simulink model "PizzaBox"  (R2018b)
settings: Solver=FixedStepAuto  StartTime=0.0  StopTime=inf  RelTol=1e-3  EnableMultiTasking=on
undefined symbols (not defined in the file or in its folder): dev, Main, pwm_output0
libraries: aerolibutil x7, px4Sensorslib x4, px4uORBlib x3, simulink x2, px4lib x1, sharedtransform x1
(part 1 of 2)
settings Model: xpc_rtwmakecfg_data=_xpcnblib_  SimulationMode=external  ExtModeTrigDuration=10  Creator=Robert  LastModifiedBy=Robert
settings SolverCC: PositivePriorityOrder=on
settings DataIOCC: SaveOutput=off  SignalLogging=off  DSMLogging=off  SaveTime=off
settings OptimizationCC: DefaultUnderspecifiedDataType=single  EnhancedBackFolding=on  PassReuseOutputArgsAs=Individual arguments  MaxStackSize=64  OptimizeBlockOrder=speed  DifferentSizesBufferReuse=on  OptimizationCustomize=off
settings DebuggingCC: ParameterTunabilityLossMsg=error
settings HardwareCC: ProdBitPerPointer=32  ProdBitPerSizeT=32  ProdBitPerPtrDiffT=32  ProdLargestAtomicInteger=Long  ProdLargestAtomicFloat=Double  ProdWordSize=32  ProdLongLongMode=on  ProdHWDeviceType=ARM Compatible->ARM Cortex
settings SFSimCC: MATLABDynamicMemAlloc=off
settings RTWCC: SystemTargetFile=ert.tlc  HardwareBoard=PX4 Pixhawk 1  TLCOptions="-aInlineSetEventsForThisBaseRateFcn=TLC_FALSE -aSuppressMultiTaskScheduler=TLC_FALSE  -aRateBasedStepFcn=0"  TemplateMakefile=ert_default_tmf  GenerateReport=on  Toolchain=GNU Tools for PX4 Autopilots  IncludeHyperlinkInReport=on  LaunchReport=on  TargetLang=C++  GenerateTraceInfo=on  GenerateTraceReport=on  GenerateTraceReportSl=on  GenerateTraceReportSf=on  GenerateTraceReportEml=on
settings CodeAppCC: ForceParamTrailComments=on  IgnoreCustomStorageClasses=off  OperatorAnnotations=on  SimulinkDataObjDesc=on  SFDataObjDesc=on  InsertBlockDesc=on
settings ERTTargetCC: ExtMode=on  ExtModeMexArgs='127.0.0.1' 1 17725

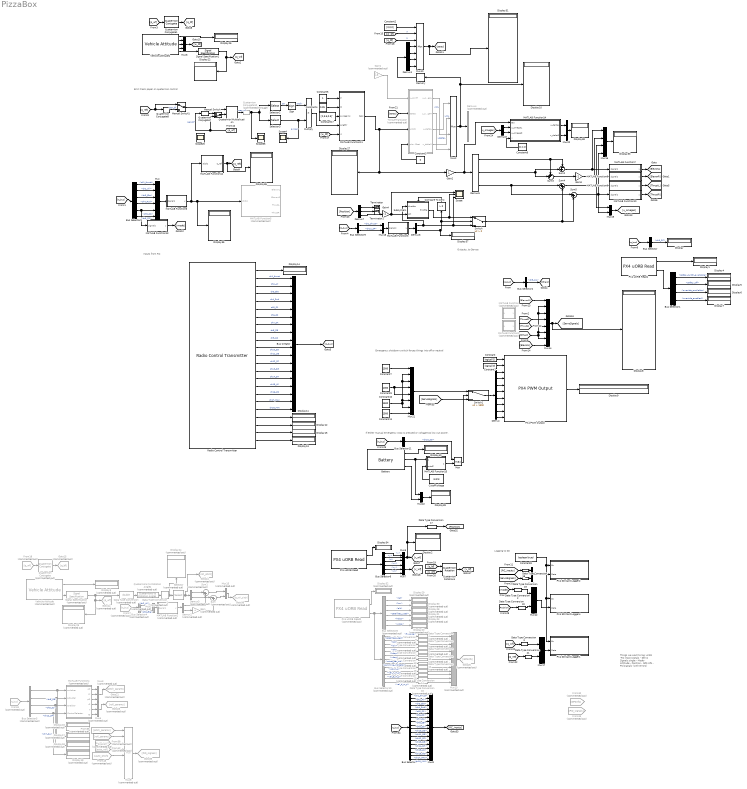
== system PizzaBox ==
  note: If either manual emergency stop is pressed or voltage too low cut power.
  note: Emergency shutdown switch forces things into
      | off or neutral
  note: Logging to SD
  note: Inputs from RC
  note: Outputs, to Servos
  note: Things we want to log:
      |
      | uint8
      | -RC input signals
      | - Servo Signals
      |
      | single
      | - Mode
      | - Attitude
      | - Position
      | - GPS info
      | - Pid signals (with errors)
  note: Emil Fresk paper on quaternion control
  Battery : px4Sensorslib/Battery  voltage=on  current=off  remaining=on  warning=off  timestamp=off  sampleTime=1/250  BlockingMode=off  BlockTimeout=1e-3
      settings: SourceProductName=Embedded Coder Support Package for PX4 Autopilots
  Bus Creator : BusCreator  Inputs=18
  Bus Selector : BusSelector  OutputSignals=ch9_SC
  Bus Selector1 : BusSelector  OutputSignals=safety_switch_available,safety_off,override_available,override_enabled
  Bus Selector10 : BusSelector  Commented=on  OutputSignals=fix_type,satellites_used,lat,lon,alt,hdop,vdop,noise_per_ms,jamming_indicator,vel_m_s,vel_n_m_s,vel_e_m_s,vel_d_m_s
  Bus Selector11 : BusSelector  OutputSignals=ch10_SD
  Bus Selector2 : BusSelector  OutputSignals=ch5_S1
  Bus Selector3 : BusSelector  OutputSignals=ch1_thrust,ch2_Ail,ch3_Ele,ch4_Rud,ch9_SC,ch6_S2
  Bus Selector4 : BusSelector  Commented=on  OutputSignals=ch2_Ail,ch3_Ele
  Bus Selector5 : BusSelector  Commented=on  OutputSignals=ch8_SB,ch5_S1,ch12_SF,ch7_SA
  Bus Selector6 : BusSelector  OutputSignals=x,y,z,vx,vy,vz
  Bus Selector7 : BusSelector  OutputSignals=ch1_thrust,ch2_Ail,ch3_Ele,ch4_Rud,ch5_S1,ch6_S2,ch7_SA,ch8_SB,ch9_SC,ch10_SD,ch11_SE,ch12_SF,ch13_SG,ch14_SH,ch15_LS,ch16_RS,ch17_MAX,ch18_MIN
  Bus Selector8 : BusSelector  Commented=on  OutputSignals=lat,lon,alt,satellites_used,hdop,vdop
  Bus Selector9 : BusSelector  OutputSignals=ch1_thrust,ch12_SF
  Compare To Zero : simulink/Logic and Bit Operations/Compare To Zero  relop=>  OutDataTypeStr=boolean
  Constant : Constant  Value=logical(1)
  Constant1 : Constant  Value=logical(0)
  Constant10 : Constant  Value=1500  OutDataTypeStr=uint16
  Constant11 : Constant  Value=1500  OutDataTypeStr=uint16
  Constant17 : Constant  Value=[2,3.5,0.3]'  VectorParams1D=off
  Constant2 : Constant  Value=[0,0,0]  OutDataTypeStr=single
  Constant3 : Constant  Value=0
  Constant4 : Constant  Value=0.25
  Constant5 : Constant
  Constant6 : Constant  Value=[0,0,0]
  Constant7 : Constant  Value=1500  OutDataTypeStr=uint16
  Constant8 : Constant  Value=boolean(true)  OutDataTypeStr=boolean  SampleTime=0.004
  Constant9 : Constant  Value=1000  OutDataTypeStr=uint16
  CutoffVoltage : Constant  Value=3.3*3  OutDataTypeStr=single
  Data Type Conversion : DataTypeConversion  Commented=on  OutDataTypeStr=double
  Data Type Conversion{1,4..16} (14 alike) : DataTypeConversion  Commented=on  OutDataTypeStr=single
  Data Type Conversion{2..3,17,20..21} (5 alike) : DataTypeConversion  OutDataTypeStr=single
  Data Type Conversion18 : DataTypeConversion  OutDataTypeStr=uint16
  Data Type Conversion19 : DataTypeConversion  OutDataTypeStr=uint16
  Demux : Demux  Outputs=8
  Demux1 : Demux
  Demux2 : Demux  Commented=on  Outputs=2
  Demux3 : Demux  Commented=on  Outputs=2
  Demux4 : Demux  Commented=on
  Demux5 : Demux  Outputs=3
  Demux6 : Demux  Outputs=2
  Demux7 : Demux  Outputs=3
  Demux8 : Demux  Outputs=2
  Display{,1..2,4..15,22,26..27,31,33..40} (27 alike) : Display
      Display9 settings: Format=binary (Stored Integer)
  Display{3,16..21,23..25,28..30,32} (14 alike) : Display  Commented=on
  From18 : From  Commented=on  GotoTag=q_wf
  From30 : From  Commented=on  GotoTag=GPSinfo
  From33 : From  Commented=on  GotoTag=PID_signals
  From36 : From  Commented=on  GotoTag=pitch_params
  From37 : From  Commented=on  GotoTag=roll_params
  From38 : From  Commented=on  GotoTag=e_roll_pitch
  From42 : From  Commented=on  GotoTag=auto_roll
  From43 : From  Commented=on  GotoTag=auto_pitch
  From7 : From  Commented=on  GotoTag=rc_bus
  From8 : From  Commented=on  GotoTag=rc_bus
  Gain : Gain  Commented=on  Gain=-1
  Gain1 : Gain  Commented=on  Gain=18
  Gain2 : Gain
  Gain3 : Gain  Gain=-1
  Gain4 : Gain  Gain=-1
  Goto14 : Goto  Commented=on  GotoTag=q_wf
  Goto15 : Goto  Commented=on  GotoTag=q_bf
  Goto21 : Goto  Commented=on  GotoTag=pitch_params
  Goto23 : Goto  Commented=on  GotoTag=roll_params
  Goto24 : Goto  Commented=on  GotoTag=roll_pitch
  Goto25 : Goto  Commented=on  GotoTag=GPSinfo
  Goto35 : Goto  Commented=on  GotoTag=PID_signals
  Goto36 : Goto  Commented=on  GotoTag=e_roll_pitch
  MATLAB Function : MATLAB Function  Commented=on  TreatAsAtomicUnit=on
  MATLAB Function1 : MATLAB Function  Commented=on  TreatAsAtomicUnit=on
  MATLAB Function10 : MATLAB Function  TreatAsAtomicUnit=on
  MATLAB Function11 : MATLAB Function  TreatAsAtomicUnit=on
  MATLAB Function12 : MATLAB Function  TreatAsAtomicUnit=on
  MATLAB Function13 : MATLAB Function  TreatAsAtomicUnit=on
  MATLAB Function14 : MATLAB Function  TreatAsAtomicUnit=on
  MATLAB Function15 : MATLAB Function  TreatAsAtomicUnit=on
  MATLAB Function2 : MATLAB Function  Commented=on  TreatAsAtomicUnit=on
  MATLAB Function3 : MATLAB Function  TreatAsAtomicUnit=on
  MATLAB Function4 : MATLAB Function  Commented=on  TreatAsAtomicUnit=on
  MATLAB Function5 : MATLAB Function  Commented=on  TreatAsAtomicUnit=on
  MATLAB Function6 : MATLAB Function  TreatAsAtomicUnit=on
  MATLAB Function7 : MATLAB Function  TreatAsAtomicUnit=on
  MATLAB Function8 : MATLAB Function  TreatAsAtomicUnit=on
  MATLAB Function9 : MATLAB Function  TreatAsAtomicUnit=on
  Manual Switch : ManualSwitch  CurrentSetting=0
  Manual Switch1 : ManualSwitch
  Max : MinMax  Function=max  Inputs=2  OutDataTypeStr=uint16
  Memory : Memory
  Multiply : Product
  Mux : Mux  Inputs=6
  Mux1 : Mux  Commented=on  Inputs=2
  Mux10 : Mux  Inputs=7
  Mux{11..12,17..20,22} (7 alike) : Mux  Inputs=2
  Mux13 : Mux  Commented=on  Inputs=13
  Mux14 : Mux  Inputs=8
  Mux15 : Mux  Commented=on  Inputs=2
  Mux16 : Mux
  Mux2 : Mux
  Mux21 : Mux  Inputs=8
  Mux3 : Mux  Commented=on  Inputs=3
  Mux4 : Mux  Commented=on  Inputs=3
  Mux5 : Mux  Inputs=3
  Mux6 : Mux  Inputs=3
  Mux7 : Mux  Inputs=3
  Mux8 : Mux  Inputs=18
  Mux9 : Mux  Commented=on  Inputs=8
  PX4 PWM Output : px4lib/PX4 PWM Output  pwmDevice=Main (/dev/pwm_output0)  pwmChannel1_=on  pwmChannel2_=on  pwmChannel3_=on  pwmChannel4_=on  pwmChannel5_=on  pwmChannel6_=on  pwmChannel7_=on  pwmChannel8_=on  forceTerminateFailsafe=off  outputErrorStatus=on
      settings: SourceProductName=Embedded Coder Support Package for PX4 Autopilots
  PX4 SD Card Logger1 : Subsystem  mask(PX4 SD Card Logger){logfile=/fs/microsd/log, logfilename=qlogs, cacheflag=off, numRecs=250*60*60}
      mask prompts: logfile "Log Folder"; logfilename "Log File Name"; cacheflag "Cache in Memory"; numRecs "Maximum Record Count"
      mask help:
      | Log data to a specified file on the SD card
      |
      | The block accepts two inputs, enable and data. The incoming data is logged into the SD card when the enable signal is high and the number of data points logged is less than the Maximum Record Count specified.
      |
      | The specified folder should be present in the SD card for logging.
      |
      | If Cache in Memory is unchecked, the data is written to the SD card at every timestep.  If Cache in Memory is checked, data is cached in the memory and is written to SD card only when enable goes low or when the number of data points logged reaches the Maximum Record Count specified.
      mask init:
      | logname=uint8([logfile,'/',logfilename]);
      mask Help: eval('codertarget.internal.helpView(''px4'',''px4sdcardexample'')');
      mask Display:
      | fprintf([get_param(gcb,'logfile'),'/',get_param(gcb,'logfilename')])
      | port_label('input',1,'en')
      | port_label('input',2,'data')
  PX4 SD Card Logger2 : Subsystem  mask(PX4 SD Card Logger){logfile=/fs/microsd/log, logfilename=rc_and_servosignals, cacheflag=off, numRecs=250*60*60}
      mask prompts: logfile "Log Folder"; logfilename "Log File Name"; cacheflag "Cache in Memory"; numRecs "Maximum Record Count"
      mask help:
      | Log data to a specified file on the SD card
      |
      | The block accepts two inputs, enable and data. The incoming data is logged into the SD card when the enable signal is high and the number of data points logged is less than the Maximum Record Count specified.
      |
      | The specified folder should be present in the SD card for logging.
      |
      | If Cache in Memory is unchecked, the data is written to the SD card at every timestep.  If Cache in Memory is checked, data is cached in the memory and is written to SD card only when enable goes low or when the number of data points logged reaches the Maximum Record Count specified.
      mask init:
      | logname=uint8([logfile,'/',logfilename]);
      mask Help: eval('codertarget.internal.helpView(''px4'',''px4sdcardexample'')');
      mask Display:
      | fprintf([get_param(gcb,'logfile'),'/',get_param(gcb,'logfilename')])
      | port_label('input',1,'en')
      | port_label('input',2,'data')
  PX4 SD Card Logger4 : Subsystem  mask(PX4 SD Card Logger){logfile=/fs/microsd/log, logfilename=MainLog, cacheflag=off, numRecs=250*60*60}
      mask prompts: logfile "Log Folder"; logfilename "Log File Name"; cacheflag "Cache in Memory"; numRecs "Maximum Record Count"
      mask help:
      | Log data to a specified file on the SD card
      |
      | The block accepts two inputs, enable and data. The incoming data is logged into the SD card when the enable signal is high and the number of data points logged is less than the Maximum Record Count specified.
      |
      | The specified folder should be present in the SD card for logging.
      |
      | If Cache in Memory is unchecked, the data is written to the SD card at every timestep.  If Cache in Memory is checked, data is cached in the memory and is written to SD card only when enable goes low or when the number of data points logged reaches the Maximum Record Count specified.
      mask init:
      | logname=uint8([logfile,'/',logfilename]);
      mask Help: eval('codertarget.internal.helpView(''px4'',''px4sdcardexample'')');
      mask Display:
      | fprintf([get_param(gcb,'logfile'),'/',get_param(gcb,'logfilename')])
      | port_label('input',1,'en')
      | port_label('input',2,'data')
  PX4 uORB Read : px4uORBlib/PX4 uORB Read  uORBTopic=vehicle_local_position  sampleTime=0.004  BlockingMode=off  BlockTimeout=1e-3
      settings: SourceProductName=Embedded Coder Support Package for PX4 Autopilots
  PX4 uORB Read1 : px4uORBlib/PX4 uORB Read  uORBTopic=safety  sampleTime=0.004  BlockingMode=off  BlockTimeout=1e-3
      settings: SourceProductName=Embedded Coder Support Package for PX4 Autopilots
  PX4 uORB Read2 : px4uORBlib/PX4 uORB Read  Commented=on  uORBTopic=vehicle_gps_position  sampleTime=0.004  BlockingMode=off  BlockTimeout=1e-3
      settings: SourceProductName=Embedded Coder Support Package for PX4 Autopilots
  Quaternion Conjugate : aerolibutil/Quaternion Conjugate  Commented=on
      settings: SourceProductName=Aerospace Blockset  SourceProductBaseCode=AE
  Quaternion Conjugate1 : aerolibutil/Quaternion Conjugate
      settings: SourceProductName=Aerospace Blockset  SourceProductBaseCode=AE
  Quaternion Conjugate10 : aerolibutil/Quaternion Conjugate  Commented=through
      settings: SourceProductName=Aerospace Blockset  SourceProductBaseCode=AE
  Quaternion Conjugate7 : aerolibutil/Quaternion Conjugate
      settings: SourceProductName=Aerospace Blockset  SourceProductBaseCode=AE
  Quaternion Conjugate8 : aerolibutil/Quaternion Conjugate
      settings: SourceProductName=Aerospace Blockset  SourceProductBaseCode=AE
  Quaternion Multiplication : aerolibutil/Quaternion Multiplication
  Quaternion Rotation4 : aerolibutil/Quaternion Rotation
  Quaternions to Rotation Angles : sharedtransform/Quaternions to Rotation Angles  Commented=on  rotationOrder=ZYX  aMode=aMode
      settings: SourceProductBaseCode=AE
  Radio Control Transmitter : px4Sensorslib/Radio Control Transmitter  channel1=on  channel2=on  channel3=on  channel4=on  channel5=on  channel6=on  channel7=on  channel8=on  channel9=on  channel10=on  channel11=on  channel12=on  channel13=on  channel14=on  channel15=on  channel16=on  channel17=on  channel18=on  channel_count=on  rssi=on  rc_input_source=on  timestamp_last_signal=on  time_stamp=off  sampleTime=1/250  BlockingMode=off  BlockTimeout=5
      settings: SourceProductName=Embedded Coder Support Package for PX4 Autopilots
  Scope : Scope  NumInputPorts=3
  Scope25 : Scope
  Scope35 : Scope
  Scope4 : Scope
  Selector : Selector  Commented=on  InputPortWidth=3  IndexOptions=Index vector (dialog)  Indices=[3 2]  OutputSizes=1
  Selector2 : Selector  IndexMode=Zero-based  InputPortWidth=4  IndexOptions=Index vector (dialog)  Indices=[0 ]  OutputSizes=1
  Selector3 : Selector  IndexMode=Zero-based  InputPortWidth=4  IndexOptions=Index vector (dialog)  Indices=[1:3]  OutputSizes=1
  Sign : Signum
  Signal Specification : SignalSpecification  Commented=on  OutDataTypeStr=single
  Signal Specification1 : SignalSpecification  OutDataTypeStr=single
  Subsystem : Subsystem
  Sum : Sum  Commented=on  Inputs=|-+
  Sum1 : Sum  Commented=on  Inputs=|-+
  Sum2 : Sum  Inputs=-+|
  Sum3 : Sum  Inputs=++|
  Sum4 : Sum  Inputs=|++
  Sum5 : Sum  Inputs=|-+
  Switch : Switch  Criteria=u2 > Threshold
  Switch1 : Switch  Criteria=u2 > Threshold  Threshold=1300
  Terminator : Terminator
  Terminator1 : Terminator
  TorqueTranslator : MATLAB Function  Commented=on  TreatAsAtomicUnit=on
  Vehicle Attitude : px4Sensorslib/Vehicle Attitude  Commented=on  rollRate=off  pitchRate=off  yawRate=off  quaternion=on  uorbTimeStamp=off  BlockingMode=off  BlockTimeout=0.001  sampleTime=1/250
      settings: SourceProductName=Embedded Coder Support Package for PX4 Autopilots
  Vehicle Attitude1 : px4Sensorslib/Vehicle Attitude  rollRate=on  pitchRate=on  yawRate=on  quaternion=on  uorbTimeStamp=off  BlockingMode=off  BlockTimeout=0.001  sampleTime=1/250
      settings: SourceProductName=Embedded Coder Support Package for PX4 Autopilots
  wires:
  Vehicle Attitude/2 -> Signal Specification/1
  Vehicle Attitude/1 -> Display3/1
  Radio Control Transmitter/8 -> Bus Creator/7  "ch7_SA"
  Radio Control Transmitter/7 -> Bus Creator/6  "ch6_S2"
  Radio Control Transmitter/6 -> Bus Creator/5  "ch5_S1"
  Radio Control Transmitter/2 -> Bus Creator/1  "ch1_thrust"
  Radio Control Transmitter/3 -> Bus Creator/2  "ch2_Ail"
  Radio Control Transmitter/4 -> Bus Creator/3  "ch3_Ele"
  Radio Control Transmitter/5 -> Bus Creator/4  "ch4_Rud"
  Radio Control Transmitter/9 -> Bus Creator/8  "ch8_SB"
  Radio Control Transmitter/20 -> Display11/1
  Radio Control Transmitter/21 -> Display12/1
  Radio Control Transmitter/23 -> Display13/1
  Radio Control Transmitter/1 -> Display14/1
  Radio Control Transmitter/22 -> Display15/1
  Constant/1 -> PX4 PWM Output/1
  Constant1/1 -> PX4 PWM Output/2
  Bus Creator/1 -> [rc_bus]
  Quaternions to Rotation Angles/1 -> Data Type Conversion1/1
  Bus Selector/1 -> Display/1  "<ch9_SC>"
  Demux3/1 -> Sum1/1
  Demux3/2 -> Sum/1
  Signal Specification/1 -> Goto14/1, Display25/1, Data Type Conversion/1
  [rc_bus] -> Bus Selector2/1
  [rc_bus] -> Bus Selector/1
  Bus Selector2/1 -> [Others]  "<ch5_S1>"
  Data Type Conversion/1 -> Quaternions to Rotation Angles/1
  Demux2/2 -> Gain/1
  From7/1 -> Bus Selector4/1
  Bus Selector4/1 -> Mux1/1  "<ch2_Ail>"
  Bus Selector4/2 -> Mux1/2  "<ch3_Ele>"
  Mux1/1 -> MATLAB Function2/1(signals)
  MATLAB Function2/1(y) -> Demux2/1
  Demux2/1 -> Sum1/2
  Mux4/1 -> Goto23/1
  From8/1 -> Bus Selector5/1
  Bus Selector5/2 -> Display17/1, MATLAB Function4/2(adjuster)  "<ch5_S1>"
  Bus Selector5/1 -> Display16/1, MATLAB Function4/1(switcher)  "<ch8_SB>"
  MATLAB Function4/1(pP) -> Mux3/1
  MATLAB Function4/2(pI) -> Mux3/2
  MATLAB Function4/3(pD) -> Mux3/3
  Bus Selector5/3 -> Display18/1, MATLAB Function4/3(enabler)  "<ch12_SF>"
  Radio Control Transmitter/10 -> Bus Creator/9  "ch9_SC"
  Radio Control Transmitter/11 -> Bus Creator/10  "ch10_SD"
  Radio Control Transmitter/12 -> Bus Creator/11  "ch11_SE"
  Radio Control Transmitter/13 -> Bus Creator/12  "ch12_SF"
  Radio Control Transmitter/14 -> Bus Creator/13  "ch13_SG"
  Radio Control Transmitter/15 -> Bus Creator/14  "ch14_SH"
  Radio Control Transmitter/16 -> Bus Creator/15  "ch15_LS"
  Radio Control Transmitter/17 -> Bus Creator/16  "ch16_RS"
  Radio Control Transmitter/18 -> Bus Creator/17  "ch17_MAX"
  Radio Control Transmitter/19 -> Bus Creator/18  "ch18_MIN"
  MATLAB Function4/4(rP) -> Mux4/1
  MATLAB Function4/5(rI) -> Mux4/2
  MATLAB Function4/6(rD) -> Mux4/3
  Bus Selector5/4 -> Display19/1, MATLAB Function4/4(ControlSelector)  "<ch7_SA>"
  PX4 uORB Read/2 -> Bus Selector6/1
  PX4 uORB Read2/2 -> Bus Selector10/1, Bus Selector8/1
  PX4 uORB Read/1 -> Display34/1
  PX4 uORB Read2/1 -> Display32/1
  Bus Selector6/1 -> Mux5/1  "<x>"
  Bus Selector6/2 -> Mux5/2  "<y>"
  Bus Selector6/3 -> Mux5/3  "<z>"
  Bus Selector8/1 -> Display29/1  "<lat>"
  Bus Selector8/2 -> Display30/1  "<lon>"
  Bus Selector8/3 -> Display28/1  "<alt>"
  Sum1/1 -> Mux15/1
  Sum/1 -> Mux15/2
  Gain/1 -> Sum/2
  Mux3/1 -> Goto21/1
  Selector/1 -> Goto24/1, Demux3/1
  Mux5/1 -> Data Type Conversion17/1, Display2/1, [r_wf]
  From18/1 -> Quaternion Conjugate/1
  Quaternion Conjugate/1 -> Goto15/1
  Bus Selector6/4 -> Mux7/1  "<vx>"
  Bus Selector6/5 -> Mux7/2  "<vy>"
  Bus Selector6/6 -> Mux7/3  "<vz>"
  Mux7/1 -> [v_wf]
  Quaternion Rotation4/1 -> [v_bf]
  [v_wf] -> Quaternion Rotation4/2
  [q_bf] -> Quaternion Rotation4/1
  Bus Selector8/4 -> Display21/1  "<satellites_used>"
  Bus Selector8/5 -> Display23/1  "<hdop>"
  Bus Selector8/6 -> Display20/1  "<vdop>"
  Data Type Conversion1/1 -> Display24/1, Selector/1
  Constant8/1 -> PX4 SD Card Logger1/1(En), PX4 SD Card Logger4/1(En), PX4 SD Card Logger2/1(En)
  Mux11/1 -> PX4 SD Card Logger2/2(Data)
  [RC_inputs] -> Data Type Conversion18/1
  [ServoSignals] -> Data Type Conversion19/1
  Mux12/1 -> PX4 SD Card Logger4/2(Data)
  [mode] -> Data Type Conversion2/1
  [Position] -> Data Type Conversion20/1
  Bus Selector10/1 -> Data Type Conversion4/1  "<fix_type>"
  Bus Selector10/2 -> Data Type Conversion5/1  "<satellites_used>"
  Bus Selector10/3 -> Data Type Conversion6/1  "<lat>"
  Bus Selector10/4 -> Data Type Conversion7/1  "<lon>"
  Bus Selector10/5 -> Data Type Conversion8/1  "<alt>"
  Bus Selector10/6 -> Data Type Conversion9/1  "<hdop>"
  Bus Selector10/7 -> Data Type Conversion10/1  "<vdop>"
  Bus Selector10/8 -> Data Type Conversion11/1  "<noise_per_ms>"
  Bus Selector10/9 -> Data Type Conversion12/1  "<jamming_indicator>"
  Bus Selector10/10 -> Data Type Conversion13/1  "<vel_m_s>"
  Bus Selector10/11 -> Data Type Conversion14/1  "<vel_n_m_s>"
  Bus Selector10/12 -> Data Type Conversion15/1  "<vel_e_m_s>"
  Bus Selector10/13 -> Data Type Conversion16/1  "<vel_d_m_s>"
  Mux13/1 -> Goto25/1
  [rc_bus] -> Bus Selector7/1
  Bus Selector7/1 -> Mux8/1  "<ch1_thrust>"
  Bus Selector7/2 -> Mux8/2  "<ch2_Ail>"
  Bus Selector7/3 -> Mux8/3  "<ch3_Ele>"
  Bus Selector7/4 -> Mux8/4  "<ch4_Rud>"
  Bus Selector7/5 -> Mux8/5  "<ch5_S1>"
  Bus Selector7/6 -> Mux8/6  "<ch6_S2>"
  Bus Selector7/7 -> Mux8/7  "<ch7_SA>"
  Bus Selector7/8 -> Mux8/8  "<ch8_SB>"
  Bus Selector7/9 -> Mux8/9  "<ch9_SC>"
  Bus Selector7/10 -> Mux8/10  "<ch10_SD>"
  Bus Selector7/11 -> Mux8/11  "<ch11_SE>"
  Bus Selector7/12 -> Mux8/12  "<ch12_SF>"
  Bus Selector7/13 -> Mux8/13  "<ch13_SG>"
  Bus Selector7/14 -> Mux8/14  "<ch14_SH>"
  Bus Selector7/15 -> Mux8/15  "<ch15_LS>"
  Bus Selector7/16 -> Mux8/16  "<ch16_RS>"
  Bus Selector7/17 -> Mux8/17  "<ch17_MAX>"
  Bus Selector7/18 -> Mux8/18  "<ch18_MIN>"
  Mux8/1 -> [RC_inputs]
  Mux14/1 -> Display8/1, [ServoSignals]
  Demux/1 -> PX4 PWM Output/3
  Demux/2 -> PX4 PWM Output/4
  Demux/3 -> PX4 PWM Output/5
  Demux/4 -> PX4 PWM Output/6
  Demux/5 -> PX4 PWM Output/7
  Demux/6 -> PX4 PWM Output/8
  Demux/7 -> PX4 PWM Output/9
  Demux/8 -> PX4 PWM Output/10
  Mux9/1 -> Goto35/1
  From36/1 -> Mux9/1
  From37/1 -> Mux9/2
  Mux15/1 -> Goto36/1
  From38/1 -> Mux9/3
  Data Type Conversion4/1 -> Mux13/1
  Data Type Conversion5/1 -> Mux13/2
  Data Type Conversion6/1 -> Mux13/3
  Data Type Conversion7/1 -> Mux13/4
  Data Type Conversion8/1 -> Mux13/5
  Data Type Conversion9/1 -> Mux13/6
  Data Type Conversion10/1 -> Mux13/7
  Data Type Conversion11/1 -> Mux13/8
  Data Type Conversion12/1 -> Mux13/9
  Data Type Conversion13/1 -> Mux13/10
  Data Type Conversion14/1 -> Mux13/11
  Data Type Conversion15/1 -> Mux13/12
  Data Type Conversion16/1 -> Mux13/13
  Data Type Conversion17/1 -> [Position]
  Data Type Conversion18/1 -> Mux11/1
  Data Type Conversion19/1 -> Mux11/2
  From42/1 -> Mux9/4
  From43/1 -> Mux9/5
  [ThrustR] -> Mux14/4
  [ThrustL] -> Mux14/5
  [ElevonR] -> Mux14/1
  [ElevonL] -> Mux14/8
  [Others] -> Mux14/2, Mux14/3, Mux14/6, Mux14/7
  [rc_bus] -> Bus Selector3/1
  Bus Selector3/4 -> Mux/4  "<ch4_Rud>"
  Bus Selector3/1 -> Mux/1  "<ch1_thrust>"
  Bus Selector3/3 -> Mux/3  "<ch3_Ele>"
  Bus Selector3/2 -> Mux/2  "<ch2_Ail>"
  Mux/1 -> MATLAB Function6/1(signals)
  MATLAB Function6/1(y) -> MATLAB Function12/1(sticks), Display35/1, MATLAB Function5/1(sticks)
  MATLAB Function7/1(y) -> [ElevonL]
  MATLAB Function8/1(y) -> [ElevonR]
  MATLAB Function9/1(y) -> [ThrustL]
  MATLAB Function10/1(y) -> [ThrustR]
  PX4 uORB Read1/1 -> Display1/1
  PX4 uORB Read1/2 -> Bus Selector1/1
  Bus Selector1/1 -> Display4/1  "<safety_switch_available>"
  Bus Selector1/2 -> Display5/1  "<safety_off>"
  Bus Selector1/3 -> Display6/1  "<override_available>"
  Bus Selector1/4 -> Display7/1  "<override_enabled>"
  PX4 PWM Output/1 -> Display9/1
  Signal Specification1/1 -> [q_wf], Display22/1
  [q_wf] -> Quaternion Conjugate1/1
  Quaternion Conjugate1/1 -> [q_bf]
  Vehicle Attitude1/1 -> Display26/1
  Vehicle Attitude1/5 -> Signal Specification1/1
  Vehicle Attitude1/2 -> Mux6/1
  Vehicle Attitude1/3 -> Mux6/2
  Vehicle Attitude1/4 -> Mux6/3
  Mux6/1 -> [w_bf]
  Sign/1 -> Multiply/1  "rotdir"
  [w_bf] -> MATLAB Function11/5(w)
  Quaternion Multiplication/1 -> Quaternion Conjugate10/1  "qerr_wf"
  Quaternion Conjugate10/1 -> Selector3/1, Selector2/1, Scope35/1
  Constant17/1 -> MATLAB Function11/3(axisgains)
  Selector3/1 -> Multiply/2, Scope4/1  "axiserr"
  [q_wf] -> Manual Switch/2, Quaternion Conjugate7/1  "qerr_bf"
  Multiply/1 -> MATLAB Function11/4(angErr)
  Selector2/1 -> Sign/1  "q0"
  [q_ref] -> Manual Switch1/1, Quaternion Conjugate8/1
  Constant2/1 -> Mux10/1
  [w_bf] -> Mux10/2  "w"
  [q_bf] -> Mux10/3  "q"
  MATLAB Function12/1(q_ref) -> Display36/1, [q_ref]
  Demux1/1 -> Mux10/4
  Demux1/2 -> Mux10/5
  Demux1/3 -> Mux10/6
  Demux1/4 -> Mux10/7
  Memory/1 -> Demux1/1
  TorqueTranslator/3(u_deltaL) -> Mux2/1  "uWL"
  TorqueTranslator/4(u_deltaR) -> Mux2/2  "udeltaL"
  TorqueTranslator/2(u_omegaR) -> Mux2/4
  TorqueTranslator/1(u_omegaL) -> Mux2/3  "uWL"
  Mux10/1 -> Display31/1, [states]
  [states] -> TorqueTranslator/2(states)
  Constant3/1 -> TorqueTranslator/4(pitchoffset)
  MATLAB Function11/1(taos) -> Gain2/1, Display27/1, TorqueTranslator/3(wdots)
  Gain1/1 -> TorqueTranslator/1(u_jointT)
  Mux2/1 -> Display10/1, Memory/1, Demux4/1
  Sum3/1 -> Gain3/1
  Sum4/1 -> Mux19/1, Mux16/3, MATLAB Function9/1(signals)
  Sum5/1 -> Mux19/2, Mux16/4, MATLAB Function10/1(signals)
  Bus Selector9/1 -> Mux18/1  "<ch1_thrust>"
  Switch/1 -> Sum4/2, Sum5/2
  [rc_bus] -> Bus Selector9/1
  Demux5/3 -> Sum5/1, Sum4/1
  Gain2/1 -> Demux5/1, MATLAB Function14/1(tao)
  Constant5/1 -> MATLAB Function11/1(P)
  Constant4/1 -> MATLAB Function11/2(D)
  Sum2/1 -> Mux16/1, MATLAB Function7/1(signals)
  Mux16/1 -> Display33/1
  Quaternion Conjugate7/1 -> Manual Switch/1
  Manual Switch/1 -> Quaternion Multiplication/2
  Quaternion Conjugate8/1 -> Manual Switch1/2  "qerr_bf"
  Manual Switch1/1 -> Quaternion Multiplication/1
  Demux5/2 -> Sum3/2, Sum2/2
  Demux5/1 -> Sum2/1, Sum3/1
  Gain3/1 -> Mux16/2, MATLAB Function8/1(signals)
  Bus Selector3/5 -> MATLAB Function13/1(signals), Mux/5  "<ch9_SC>"
  Bus Selector3/6 -> Mux/6  "<ch6_S2>"
  MATLAB Function13/1(y) -> [mode]
  Data Type Conversion2/1 -> Mux12/1
  Data Type Conversion20/1 -> Mux12/2
  [q_ref] -> Data Type Conversion21/1
  [q_wf] -> Data Type Conversion3/1
  Data Type Conversion3/1 -> Mux17/1
  Data Type Conversion21/1 -> Mux17/2
  Mux17/1 -> PX4 SD Card Logger1/2(Data)
  Bus Selector9/2 -> Mux18/2  "<ch12_SF>"
  Mux18/1 -> MATLAB Function3/1(signals)
  MATLAB Function3/1(y) -> Demux6/1
  Demux6/2 -> Display37/1, Switch/2, Compare To Zero/1
  Demux6/1 -> Subsystem/1(throttle), Scope/3, Switch/3
  [Position] -> Demux7/1
  Demux7/1 -> Terminator/1
  Demux7/2 -> Terminator1/1
  Demux7/3 -> Gain4/1
  Gain4/1 -> Scope/1, Subsystem/2(alt)
  Compare To Zero/1 -> Subsystem/Enable
  Subsystem/1("throttle ") -> Scope/2, Switch/1
  Constant6/1 -> MATLAB Function14/4(v)
  Mux19/1 -> [u_omegas]
  Demux8/1 -> MATLAB Function14/2(u_omegaL)
  Demux8/2 -> MATLAB Function14/3(u_omegaR)
  [u_omegas] -> Demux8/1
  MATLAB Function14/2(u_deltaR) -> Mux20/2
  MATLAB Function14/1(u_deltaL) -> Mux20/1
  Mux20/1 -> Display38/1
  [rc_bus] -> Bus Selector11/1
  Max/1 -> Switch1/2
  [ServoSignals] -> Switch1/3
  Constant10/1 -> Mux21/2, Mux21/3, Mux21/6, Mux21/7
  Constant9/1 -> Mux21/4, Mux21/5
  Constant11/1 -> Mux21/8
  Constant7/1 -> Mux21/1
  Mux21/1 -> Switch1/1
  Switch1/1 -> Demux/1
  MATLAB Function15/1(stopsig) -> Max/2
  Bus Selector11/1 -> Max/1  "<ch10_SD>"
  Battery/2 -> MATLAB Function15/1(voltage), Mux22/1
  Battery/3 -> Mux22/2
  Mux22/1 -> Display39/1
  Battery/1 -> Display40/1
  CutoffVoltage/1 -> MATLAB Function15/2(cutoff)

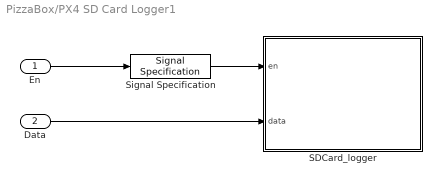
== system PizzaBox/PX4 SD Card Logger1 ==
  En : Inport
  Data : Inport  Port=2
  SDCard_logger : MATLAB Function  TreatAsAtomicUnit=on
  Signal Specification : SignalSpecification  OutDataTypeStr=boolean
  wires:
  Signal Specification/1 -> SDCard_logger/1(en)
  En/1 -> Signal Specification/1
  Data/1 -> SDCard_logger/2(data)

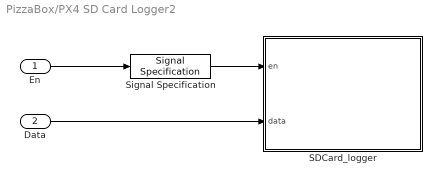
== system PizzaBox/PX4 SD Card Logger2 ==
  En : Inport
  Data : Inport  Port=2
  SDCard_logger : MATLAB Function  TreatAsAtomicUnit=on
  Signal Specification : SignalSpecification  OutDataTypeStr=boolean
  wires:
  Signal Specification/1 -> SDCard_logger/1(en)
  En/1 -> Signal Specification/1
  Data/1 -> SDCard_logger/2(data)

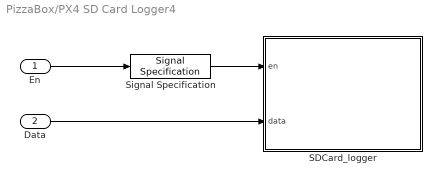
== system PizzaBox/PX4 SD Card Logger4 ==
  En : Inport
  Data : Inport  Port=2
  SDCard_logger : MATLAB Function  TreatAsAtomicUnit=on
  Signal Specification : SignalSpecification  OutDataTypeStr=boolean
  wires:
  Signal Specification/1 -> SDCard_logger/1(en)
  En/1 -> Signal Specification/1
  Data/1 -> SDCard_logger/2(data)

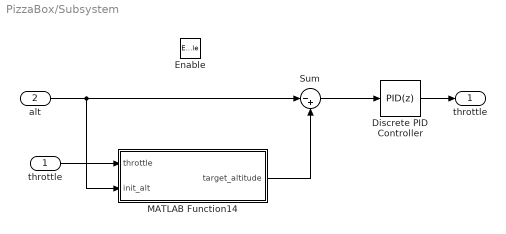
== system PizzaBox/Subsystem ==
  throttle : Inport
  alt : Inport  Port=2
  Enable : EnablePort  StatesWhenEnabling=reset
  Discrete PID Controller : simulink/Continuous/PID Controller  Controller=PID  Form=Parallel  TimeDomain=Discrete-time  SampleTime=-1  IntegratorMethod=Forward Euler  FilterMethod=Forward Euler  ControllerParametersSource=internal  P=1.5  I=0.1  D=0.5  UseFilter=off  N=100  TunerSelectOption=Transfer Function Based (PID Tuner App)  InitialConditionSource=internal  InitialConditionForIntegrator=0  InitialConditionForFilter=0  DifferentiatorICPrevScaledInput=0  ExternalReset=none  TrackingMode=off  Kt=1  LimitOutput=on  UpperSaturationLimit=1  LowerSaturationLimit=-1  LinearizeAsGain=off  AntiWindupMode=none  Kb=1  POutMin=[]  POutMax=[]  IOutMin=[]  IOutMax=[]  DOutMin=[]  DOutMax=[]  NOutMin=[]  NOutMax=[]  SumOutMin=[]  SumOutMax=[]  SaturationOutMin=[]  SaturationOutMax=[]  PParamMin=[]  PParamMax=[]  IParamMin=[]  IParamMax=[]  DParamMin=[]  DParamMax=[]  NParamMin=[]  NParamMax=[]  KbParamMin=[]  KbParamMax=[]  KtParamMin=[]  KtParamMax=[]  KbOutMin=[]  KbOutMax=[]  KtOutMin=[]  KtOutMax=[]  IntegratorOutMin=[]  IntegratorOutMax=[]  FilterOutMin=[]  FilterOutMax=[]  SumI1OutMin=[]  SumI1OutMax=[]  SumI2OutMin=[]  SumI2OutMax=[]  SumI3OutMin=[]  SumI3OutMax=[]  SumI4OutMin=[]  SumI4OutMax=[]  SumDOutMin=[]  SumDOutMax=[]  DifferentiatorOutMin=[]  DifferentiatorOutMax=[]  FilterDiffOutCoefMin=[]  FilterDiffOutCoefMax=[]  ReciprocalOutMin=[]  ReciprocalOutMax=[]  SumDenOutMin=[]  SumDenOutMax=[]  SumNumOutMin=[]  SumNumOutMax=[]  DivideOutMin=[]  DivideOutMax=[]  IntegratorContinuousStateAttributes=''  IntegratorStateMustResolveToSignalObject=off  IntegratorRTWStateStorageClass=Auto  FilterContinuousStateAttributes=''  FilterStateMustResolveToSignalObject=off  FilterRTWStateStorageClass=Auto  ParallelPVariant=InternalParameters  IdealPVariant=Disabled  IVariant=InternalParameters  DVariant=InternalParameters  IntegratorVariant=Discrete  SatVariant=Enabled  AWVariant=Passthrough  PCopyVariant=Disabled  TRVariant=Disabled  FdbkBlocksVariant=Forward  IdealPFdbkVariant=Disabled  SatFdbkVariant=Disabled  DerivativeFilterVariant=Differentiator  NVariant=Passthrough  NCopyVariant=Disabled_SignalSpec  FilterICVariant=InternalICsDifferentiator  IntegratorICVariant=InternalICs  ExternalResetVariant=Disabled  TRSumVariant=Passthrough  SumFdbkVariant=Disabled  SumVariant=Sum_PID
  MATLAB Function14 : MATLAB Function  TreatAsAtomicUnit=on
  Sum : Sum  Inputs=|-+
  "throttle " : Outport
  wires:
  throttle/1 -> MATLAB Function14/1(throttle)
  MATLAB Function14/1(target_altitude) -> Sum/2
  Sum/1 -> Discrete PID Controller/1
  Discrete PID Controller/1 -> "throttle "/1
  alt/1 -> MATLAB Function14/2(init_alt), Sum/1

== matlab function PizzaBox/MATLAB Function1 ==
  data: u input uint16; y output uint16
function y = invertpwm(u)

y = uint16(1500-(single(u)-1500));

== matlab function PizzaBox/MATLAB Function ==
  data: u input uint16; y output uint16
function y = invertpwm(u)

y = uint16(1500-(single(u)-1500));

== matlab function PizzaBox/MATLAB Function2 ==
  data: signals input uint16; y output single
function y = pwm2signal(signals)

y = single(signals);
% Shift to center
y = y-1500;
% Range is ~1000-2000, ie +-500, but in is +-1
y = y./500;

== matlab function PizzaBox/MATLAB Function3 ==
  data: signals input uint16; y output single
function y = pwm2signal(signals)

y = single(signals);
% Shift to center
y = y-1500;
% Range is ~1000-2000, ie +-500, but in is +-1
y = y./500;

== matlab function PizzaBox/MATLAB Function4 ==
  data: switcher input uint16; pP output single; adjuster input uint16; pI output single; pD output single; enabler input uint16; ControlSelector input uint16; rP output single; rI output single; rD output single
function [pP,pI,pD,rP,rI,rD] = fcn(switcher, adjuster, enabler, ControlSelector)

persistent pkP pkI pkD rkP rkI rkD;
if isempty(pkP)
    pkP = single(1);
end
if isempty(pkI)
    pkI = single(0.4);
end
if isempty(pkD)
    pkD = single(0.025);
end
if isempty(rkP)
    rkP = single(1);
end
if isempty(rkI)
    rkI = single(0.4);
end
if isempty(rkD)
    rkD = single(0.05);
end

if enabler>1500
    if ControlSelector < 1400 % Top, Roll controll
        if switcher < 1400 % Top, P
            rkP = 1+(single(adjuster)-1500)./500; 
        elseif switcher > 1600 % Bottom, D
            rkD = 0.05+0.05*(single(adjuster)-1500)./500;
        else
            rkI = 0.4+0.4*(single(adjuster)-1500)./500;
        end
    elseif ControlSelector < 1600 % Mid, Pitch control
        if switcher < 1400 % Top, P
            pkP = 1+(single(adjuster)-1500)./500; 
        elseif switcher > 1600 % Bottom, D
            pkD = 0.025+0.025*(single(adjuster)-1500)./500;
        else
            pkI = 0.4+0.4*(single(adjuster)-1500)./500;
        end
    else
        % No controller set here yet
    end
end

pP = pkP;
pI = pkI;
pD = pkD;
rP = rkP;
rI = rkI;
rD = rkD;

== matlab function PizzaBox/MATLAB Function5 ==
  data: sticks input; ElevonL output single; ElevonR output single; ThrustL output single; ThrustR output single
function [ElevonL,ElevonR,ThrustL,ThrustR] = sticks2servos(sticks)

thrust = sticks(1);
ail = sticks(2);
ele = sticks(3);
rud = sticks(4);

ElevonL = -ail-ele;
ElevonR = -ail+ele;

ThrustL = thrust+rud;
ThrustR = thrust-rud;

== matlab function PizzaBox/MATLAB Function6 ==
  data: signals input uint16; y output single
function y = pwm2signal(signals)

y = single(signals);
% Shift to center
y = y-1500;
% Range is ~1000-2000, ie +-500, but in is +-1
y = y./500;

== matlab function PizzaBox/MATLAB Function7 ==
  data: signals input; y output uint16
function y = signal2pwm(signals)

y = zeros(size(signals)); % y is hard set to uint16


% Range is ~1000-2000, ie +-500, but in is +-1
signals = signals.*500;
% Shift to center PWM
signals = signals+1500;
y = uint16(signals);

== matlab function PizzaBox/MATLAB Function8 ==
  data: signals input; y output uint16
function y = signal2pwm(signals)

y = zeros(size(signals)); % y is hard set to uint16


% Range is ~1000-2000, ie +-500, but in is +-1
signals = signals.*500;
% Shift to center PWM
signals = signals+1500;
y = uint16(signals);

== matlab function PizzaBox/MATLAB Function9 ==
  data: signals input; y output uint16
function y = signal2pwm(signals)

y = zeros(size(signals)); % y is hard set to uint16


% Range is ~1000-2000, ie +-500, but in is +-1
signals = signals.*500;
% Shift to center PWM
signals = signals+1500;
y = uint16(signals);

== matlab function PizzaBox/MATLAB Function10 ==
  data: signals input; y output uint16
function y = signal2pwm(signals)

y = zeros(size(signals)); % y is hard set to uint16


% Range is ~1000-2000, ie +-500, but in is +-1
signals = signals.*500;
% Shift to center PWM
signals = signals+1500;
y = uint16(signals);

== matlab function PizzaBox/PX4 SD Card Logger2/SDCard_logger ==
  data: en input boolean; data input; logname parameter uint8; cacheflag parameter boolean; numRecs parameter uint32
%% PX4 SD Card Logger
% Note: All data needs to be of the same type (e.g. double)
% Header information format:
%           String "MWLOG"
%           Time/Date 4 bytes (time())
%           Number of Signals per record Logged 1 byte (256 max)
%           Data Type of Signals Logged  1 byte (1-10)
%           Number of bytes per record 2 bytes (65535 max)
% This does NOT include the number of data sets logged.
% i.e. The Reader is responsible for reading until EOF.
% Steve Kuznicki
% Copyright 2018 The MathWorks, Inc.

function SDCard_logger(en, data, logname, cacheflag, numRecs)

persistent fp isflushed isopen count  elem_size vect_size datastore timestore count_prev

if coder.target('Rtw')
    
    coder.cinclude('<stdio.h>');
    coder.cinclude('<time.h>');
    
    if coder.target('Rtw')
        coder.cinclude('<drivers/drv_hrt.h>');
    end
    
    if coder.target('Rtw')
        timestamp=coder.opaque('uint64_t');
        timestamp=coder.ceval('hrt_absolute_time');
    else
        timestamp = uint64(0);
    end
    
    if isempty(count)
        count = uint32(0);
        count_prev=count;
        fp = coder.opaque('FILE*', 'NULL');
        isflushed = false;
        if cacheflag == true
            datastore = zeros(numRecs*uint32(coder.const(numel(data))), 1, 'like', data);
            timestore=uint64(zeros(numRecs, 1));
        end
        
        [elsize, eltype] = get_elem_size(data);
        elem_size = coder.const(uint16(elsize));
        elem_type = coder.const(uint8(eltype));
        vect_size = coder.const(uint8(numel(data)));
        coder.ceval('printf',['OPENING file %s vect_size %d elem_size %d numRecs %d %c' uint8(0)], ...
            [logname,'.bin', int8(0)], uint32(vect_size), uint32(elem_size), uint32(numRecs), uint8(10));
        fp = coder.ceval('fopen', [logname,'.bin', int8(0)], ['wb', int8(0)]);
        isopen = true;
        
        % Write header information here
        % header token + version
        mlStrVer = 'MWLOG';
        coder.ceval('fwrite', coder.rref(mlStrVer), uint32(1), length(mlStrVer), fp);
        % date/time
        tm = uint32(0);
        tmptr = uint32(0);
        tm = coder.ceval('time',coder.wref(tmptr));
        coder.ceval('fwrite', coder.rref(tm), uint32(4), uint32(1), fp);
        % number of elements in each record
        coder.ceval('fwrite', coder.rref(vect_size), uint32(1), uint32(1), fp);
        % data type of the elements
        coder.ceval('fwrite', coder.rref(elem_type), uint32(1), uint32(1), fp);
        % size of each record in bytes
        recSize = elem_size * uint16(vect_size);
        coder.ceval('fwrite', coder.rref(recSize), uint32(2), uint32(1), fp);
    end
    
    
    if (en && (count < numRecs))
        
        if isopen == false
            % open file in append mode
            fp = coder.ceval('fopen', [logname,'.bin', int8(0)], ['ab', int8(0)]);
            isflushed = false;
            isopen = true;
            count_prev=count;
        end
        
        % cache data in memory or use fwrite
        if cacheflag == true
            addr = (count*uint32(vect_size))+1;
            for idx = 1:vect_size
                datastore(addr) = data(idx);
                addr = addr + 1;
            end
            timestore(count+uint32(1))=uint64(timestamp);
        else
            coder.ceval('fwrite', coder.rref(data), elem_size, vect_size, fp);
            if coder.target('Rtw')
                coder.ceval('fwrite', coder.rref(timestamp), uint32(8), uint32(1), fp);
            end
        end
        count = count + uint32(1);
        
    else
        if isopen == true
            if ~isflushed
                coder.ceval('printf',['CLOSING file. count = %d %c' uint8(0)], uint32(count), uint8(10));
                if cacheflag
                    for idx=count_prev+1:count
                        for idx2=(idx-1)*double(vect_size)+1:(idx-1)*double(vect_size)+double(vect_size)
                            coder.ceval('fwrite', coder.rref(datastore(idx2)), elem_size, uint32(1), fp);
                        end
                        coder.ceval('fwrite', coder.rref(timestore(idx)), uint32(8), uint32(1), fp);
                    end
                end
                coder.ceval('fflush', fp);
                isflushed = true;
            end
            coder.ceval('fclose', fp);
        end
        isopen = false;
    end
end

% return the size of the element in bytes
    function [elem_size, dtype] = get_elem_size(data)
        switch(class(data))
            case 'double'
                elem_size = 8;
                dtype = 1;
            case 'single'
                elem_size = 4;
                dtype = 2;
            case 'int32'
                elem_size = 4;
                dtype = 3;
            case 'uint32'
                elem_size = 4;
                dtype = 4;
            case 'int16'
                elem_size = 2;
                dtype = 5;
            case 'uint16'
                elem_size = 2;
                dtype = 6;
            case 'int8'
                elem_size = 1;
                dtype = 7;
            case 'uint8'
                elem_size = 1;
                dtype = 8;
            case 'logical'
                elem_size = 1;
                dtype = 9;
            case 'embedded.fi'
                nt = numerictype(data);
                elem_size = 2^ceil(log2(ceil(nt.WordLength / 8)));
                dtype = 10;
        end
        if ~isreal(data)
            elem_size = elem_size*2;
        end
        
        elem_size = uint16(elem_size);
        dtype = uint8(dtype);
    end
end

== matlab function PizzaBox/PX4 SD Card Logger4/SDCard_logger ==
  data: en input boolean; data input; logname parameter uint8; cacheflag parameter boolean; numRecs parameter uint32
%% PX4 SD Card Logger
% Note: All data needs to be of the same type (e.g. double)
% Header information format:
%           String "MWLOG"
%           Time/Date 4 bytes (time())
%           Number of Signals per record Logged 1 byte (256 max)
%           Data Type of Signals Logged  1 byte (1-10)
%           Number of bytes per record 2 bytes (65535 max)
% This does NOT include the number of data sets logged.
% i.e. The Reader is responsible for reading until EOF.
% Steve Kuznicki
% Copyright 2018 The MathWorks, Inc.

function SDCard_logger(en, data, logname, cacheflag, numRecs)

persistent fp isflushed isopen count  elem_size vect_size datastore timestore count_prev

if coder.target('Rtw')
    
    coder.cinclude('<stdio.h>');
    coder.cinclude('<time.h>');
    
    if coder.target('Rtw')
        coder.cinclude('<drivers/drv_hrt.h>');
    end
    
    if coder.target('Rtw')
        timestamp=coder.opaque('uint64_t');
        timestamp=coder.ceval('hrt_absolute_time');
    else
        timestamp = uint64(0);
    end
    
    if isempty(count)
        count = uint32(0);
        count_prev=count;
        fp = coder.opaque('FILE*', 'NULL');
        isflushed = false;
        if cacheflag == true
            datastore = zeros(numRecs*uint32(coder.const(numel(data))), 1, 'like', data);
            timestore=uint64(zeros(numRecs, 1));
        end
        
        [elsize, eltype] = get_elem_size(data);
        elem_size = coder.const(uint16(elsize));
        elem_type = coder.const(uint8(eltype));
        vect_size = coder.const(uint8(numel(data)));
        coder.ceval('printf',['OPENING file %s vect_size %d elem_size %d numRecs %d %c' uint8(0)], ...
            [logname,'.bin', int8(0)], uint32(vect_size), uint32(elem_size), uint32(numRecs), uint8(10));
        fp = coder.ceval('fopen', [logname,'.bin', int8(0)], ['wb', int8(0)]);
        isopen = true;
        
        % Write header information here
        % header token + version
        mlStrVer = 'MWLOG';
        coder.ceval('fwrite', coder.rref(mlStrVer), uint32(1), length(mlStrVer), fp);
        % date/time
        tm = uint32(0);
        tmptr = uint32(0);
        tm = coder.ceval('time',coder.wref(tmptr));
        coder.ceval('fwrite', coder.rref(tm), uint32(4), uint32(1), fp);
        % number of elements in each record
        coder.ceval('fwrite', coder.rref(vect_size), uint32(1), uint32(1), fp);
        % data type of the elements
        coder.ceval('fwrite', coder.rref(elem_type), uint32(1), uint32(1), fp);
        % size of each record in bytes
        recSize = elem_size * uint16(vect_size);
        coder.ceval('fwrite', coder.rref(recSize), uint32(2), uint32(1), fp);
    end
    
    
    if (en && (count < numRecs))
        
        if isopen == false
            % open file in append mode
            fp = coder.ceval('fopen', [logname,'.bin', int8(0)], ['ab', int8(0)]);
            isflushed = false;
            isopen = true;
            count_prev=count;
        end
        
        % cache data in memory or use fwrite
        if cacheflag == true
            addr = (count*uint32(vect_size))+1;
            for idx = 1:vect_size
                datastore(addr) = data(idx);
                addr = addr + 1;
            end
            timestore(count+uint32(1))=uint64(timestamp);
        else
            coder.ceval('fwrite', coder.rref(data), elem_size, vect_size, fp);
            if coder.target('Rtw')
                coder.ceval('fwrite', coder.rref(timestamp), uint32(8), uint32(1), fp);
            end
        end
        count = count + uint32(1);
        
    else
        if isopen == true
            if ~isflushed
                coder.ceval('printf',['CLOSING file. count = %d %c' uint8(0)], uint32(count), uint8(10));
                if cacheflag
                    for idx=count_prev+1:count
                        for idx2=(idx-1)*double(vect_size)+1:(idx-1)*double(vect_size)+double(vect_size)
                            coder.ceval('fwrite', coder.rref(datastore(idx2)), elem_size, uint32(1), fp);
                        end
                        coder.ceval('fwrite', coder.rref(timestore(idx)), uint32(8), uint32(1), fp);
                    end
                end
                coder.ceval('fflush', fp);
                isflushed = true;
            end
            coder.ceval('fclose', fp);
        end
        isopen = false;
    end
end

% return the size of the element in bytes
    function [elem_size, dtype] = get_elem_size(data)
        switch(class(data))
            case 'double'
                elem_size = 8;
                dtype = 1;
            case 'single'
                elem_size = 4;
                dtype = 2;
            case 'int32'
                elem_size = 4;
                dtype = 3;
            case 'uint32'
                elem_size = 4;
                dtype = 4;
            case 'int16'
                elem_size = 2;
                dtype = 5;
            case 'uint16'
                elem_size = 2;
                dtype = 6;
            case 'int8'
                elem_size = 1;
                dtype = 7;
            case 'uint8'
                elem_size = 1;
                dtype = 8;
            case 'logical'
                elem_size = 1;
                dtype = 9;
            case 'embedded.fi'
                nt = numerictype(data);
                elem_size = 2^ceil(log2(ceil(nt.WordLength / 8)));
                dtype = 10;
        end
        if ~isreal(data)
            elem_size = elem_size*2;
        end
        
        elem_size = uint16(elem_size);
        dtype = uint8(dtype);
    end
end

== matlab function PizzaBox/MATLAB Function12 ==
  data: sticks input; q_ref output
function q_ref = sticks2quat(sticks)

persistent ail;
persistent ele;
persistent rud;
persistent S2;
if isempty(ail)
    ail = single(0);
end
if isempty(ele)
    ele = single(0);
end
if isempty(rud)
    rud = single(0);
end
if isempty(S2)
    S2 = single(0);
end

SC = sticks(5); % MOde selector
if SC < -0.1
    % mode hover stable
    %thrust = sticks(1);
    ail = sticks(2);
    ele = sticks(3);
    rud = sticks(4);
    
elseif SC < 0.1
    % 
else
    % Mode servo setting quat, acro?
    S2 = 0.05*(sticks(6)+1); % Sensitivity setting
    ail = ail + S2*sticks(2);
    ele = ele + S2*sticks(3);
    rud = rud + S2*sticks(4);
    
end

%ElevonL = -ail-ele;
%ElevonR = -ail+ele;
%ThrustL = thrust+rud;
%ThrustR = thrust-rud;
%{
q_init = [cos(pi/4), 0, sin(pi/4), 0];
qyaw = [q00 0 0 q03];
qpitch = [q10 0 q12 0];
qroll = [q20 q21 0 0];
q0 = quatmultiply(q_init,qyaw)
q1 = quatmultiply(q0, qpitch);
q_ref = quatmultiply(q1,qroll)'
%}

q00 = cos(-rud/2);
q03 = sin(-rud/2);
q10 = cos(ele/2);
q12 = sin(ele/2);
q20 = cos(-ail/2);
q21 = sin(-ail/2);

q_init = [cos(-pi/4), 0, sin(-pi/4), 0];
qyaw = [q00 0 0 q03];
qpitch = [q10 0 q12 0];
qroll = [q20 q21 0 0];

q0 = quatmultiply(qyaw,qpitch);
q1 = quatmultiply(q0, qroll);
q_ref = quatmultiply(q1,q_init)';

== matlab function PizzaBox/MATLAB Function13 ==
  data: signals input uint16; y output single
function y = pwm2signal(signals)

y = single(signals);
% Shift to center
y = y-1500;
% Range is ~1000-2000, ie +-500, but in is +-1
y = y./500;
